simulink model "lab2_2"  (R2019b)
settings: Solver=VariableStepAuto  StartTime=0.0  StopTime=10.0  RelTol=10e-10  AbsTol=10e-10
values from neighbouring files (symbols this model uses):
  g = 9.81    [lab2.m]
  km = 0.1    [lab2.m]
  La = 0.05    [lab2.m]
  M = 0.1    [lab2.m]
  Ra = 3    [lab2.m]
  s = tf('s')    [lab2.m]
  ubar = Ra * sqrt((g * M) / km) * ybar    [lab2.m]
  ybar = 0.1    [lab2.m]
libraries: cstblocks x1
settings Model: Creator=spencersun  LastModifiedBy=spencersun

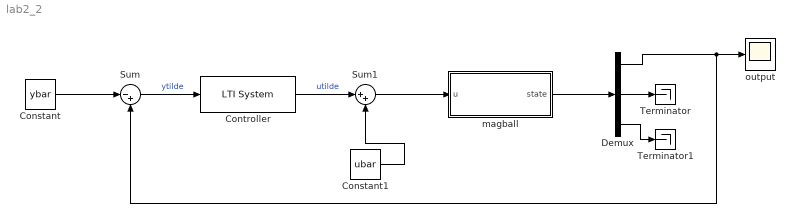
== system lab2_2 ==
  Constant : Constant  Value=ybar
  Constant1 : Constant  Value=ubar
  "Controller " : cstblocks/LTI System  sys=100*(s+10)/(s+100)  IC=[]
  Demux : Demux  Outputs=3
  Sum : Sum  Inputs=|-+
  Sum1 : Sum  Inputs=|++
  Terminator : Terminator
  Terminator1 : Terminator
  magball : Subsystem
  "output " : Scope
  wires:
  Demux/3 -> Terminator1/1
  Demux/1 -> "output "/1, Sum/2
  Demux/2 -> Terminator/1
  magball/1("state ") -> Demux/1
  "Controller "/1 -> Sum1/1  "utilde"
  Constant1/1 -> Sum1/2
  Sum1/1 -> magball/1("u ")
  Constant/1 -> Sum/1
  Sum/1 -> "Controller "/1  "ytilde"

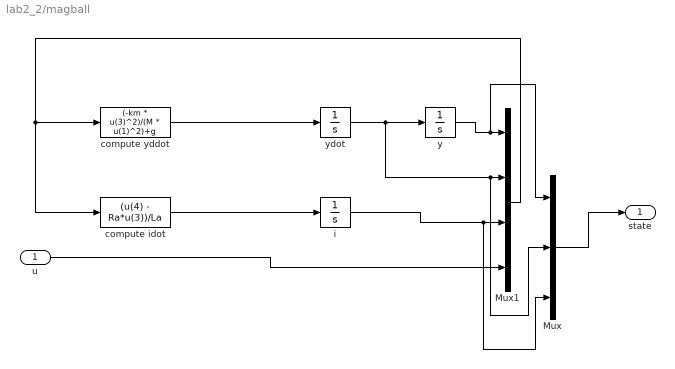
== system lab2_2/magball ==
  "u " : Inport
  Mux : Mux  Inputs=3
  Mux1 : Mux
  "compute idot " : MATLABFcn  MATLABFcn=(u(4) - Ra*u(3))/La  Output1D=off
  "compute yddot " : MATLABFcn  MATLABFcn=(-km * u(3)^2)/(M * u(1)^2)+g  Output1D=off
  "i " : Integrator
  "y " : Integrator  InitialCondition=0.15
  "ydot " : Integrator
  "state " : Outport
  wires:
  "y "/1 -> Mux/1, Mux1/1
  "ydot "/1 -> "y "/1, Mux/2, Mux1/2
  "i "/1 -> Mux/3, Mux1/3
  "u "/1 -> Mux1/4
  Mux1/1 -> "compute idot "/1, "compute yddot "/1
  "compute yddot "/1 -> "ydot "/1
  "compute idot "/1 -> "i "/1
  Mux/1 -> "state "/1
